simulink model "gm_fourxfour_designfxdpt_givens_vnl"  (R2018b)
settings: Solver=FixedStepDiscrete  StartTime=0.0  StopTime=0.18e-6  RelTol=1e-3
InitFcn:
  | if isempty(which('mylib'))
  |      tmp = fileparts(which(bdroot));
  |      run(fullfile(fileparts(tmp), '5-Utilities', 'addPathsPfcHw.m'));
  | end
  | 
  | data_types_givens
StopFcn:
  | GivensSim_Stop
undefined symbols (not defined in the file or in its folder): f
libraries: simulink x28, mylib x14
(part 3 of 4)

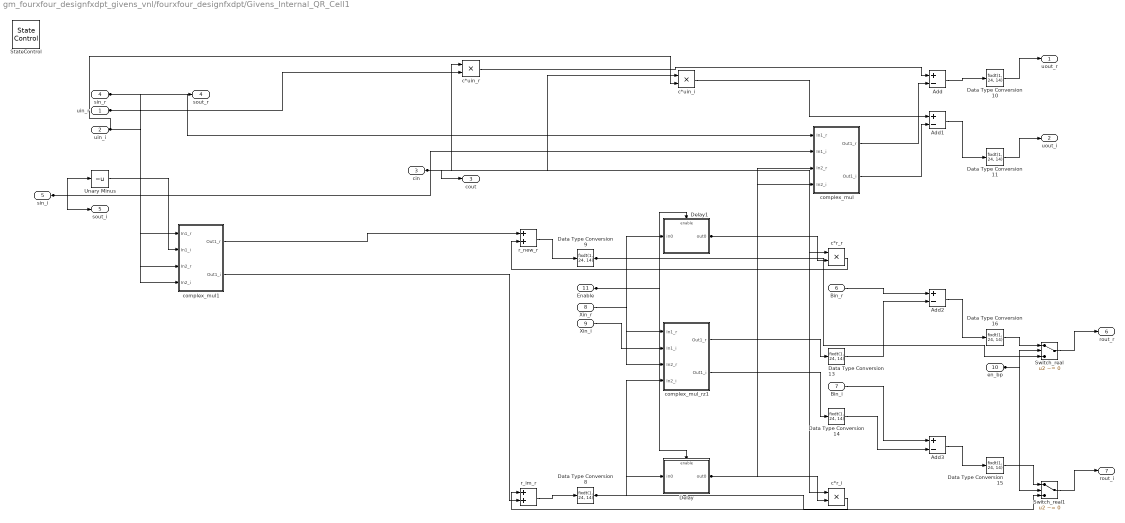
== system gm_fourxfour_designfxdpt_givens_vnl/fourxfour_designfxdpt/Givens_Internal_QR_Cell1 ==
  uin_r : Inport  OutDataTypeStr=fixdt(1, 24, 14)  SampleTime=1e-08
  uin_i : Inport  Port=2  OutDataTypeStr=fixdt(1, 24, 14)  SampleTime=1e-08
  cin : Inport  Port=3  OutDataTypeStr=fixdt(1, 24, 14)  SampleTime=1e-08
  sin_r : Inport  Port=4  OutDataTypeStr=fixdt(1, 24, 14)  SampleTime=1e-08
  sin_i : Inport  Port=5  OutDataTypeStr=fixdt(1, 24, 14)  SampleTime=1e-08
  Bin_r : Inport  Port=6  OutDataTypeStr=fixdt(1, 24, 14)  SampleTime=1e-08
  Bin_i : Inport  Port=7  OutDataTypeStr=fixdt(1, 24, 14)  SampleTime=1e-08
  Xin_r : Inport  Port=8  OutDataTypeStr=fixdt(1, 24, 14)  SampleTime=1e-08
  Xin_i : Inport  Port=9  OutDataTypeStr=fixdt(1, 24, 14)  SampleTime=1e-08
  en_bp : Inport  Port=10  OutDataTypeStr=boolean  SampleTime=1e-08
  Enable : Inport  Port=11  OutDataTypeStr=boolean  SampleTime=1e-08
  Add : Sum  Inputs=+-  AccumDataTypeStr=fixdt(1, 50, 28)  OutDataTypeStr=fixdt(1, 50, 28)  SampleTime=1e-08
  Add1 : Sum  Inputs=+-  AccumDataTypeStr=fixdt(1, 50, 28)  OutDataTypeStr=fixdt(1, 50, 28)  SampleTime=1e-08
  Add2 : Sum  Inputs=+-  AccumDataTypeStr=fixdt(1, 25, 14)  OutDataTypeStr=fixdt(1, 25, 14)  SampleTime=1e-08
  Add3 : Sum  Inputs=+-  AccumDataTypeStr=fixdt(1, 25, 14)  OutDataTypeStr=fixdt(1, 25, 14)  SampleTime=1e-08
  Data Type Conversion{8..11,13..16} (8 alike) : DataTypeConversion  OutDataTypeStr=fixdt(1, 24, 14)  SampleTime=1e-08
  Delay : Subsystem
      settings: MinAlgLoopOccurrences=on
  Delay1 : Subsystem
      settings: MinAlgLoopOccurrences=on
  StateControl : StateControl  StateControl=Synchronous
  Switch_real : Switch  Criteria=u2 ~= 0  Threshold=double(0)  OutDataTypeStr=fixdt(1, 24, 14)  SampleTime=1e-08
  Switch_real1 : Switch  Criteria=u2 ~= 0  Threshold=double(0)  OutDataTypeStr=fixdt(1, 24, 14)  SampleTime=1e-08
  Unary Minus : UnaryMinus  SampleTime=1e-08
  c*r_i : Product  Inputs=**  OutDataTypeStr=fixdt(1, 48, 28)  SampleTime=1e-08
  c*r_r : Product  Inputs=**  OutDataTypeStr=fixdt(1, 48, 28)  SampleTime=1e-08
  c*uin_i : Product  Inputs=**  OutDataTypeStr=fixdt(1, 48, 28)  SampleTime=1e-08
  c*uin_r : Product  Inputs=**  OutDataTypeStr=fixdt(1, 48, 28)  SampleTime=1e-08
  complex_mul : Subsystem
  complex_mul1 : Subsystem
  complex_mul_rz1 : Subsystem
  r_im_r : Sum  AccumDataTypeStr=fixdt(1, 50, 28)  OutDataTypeStr=fixdt(1, 50, 28)  SampleTime=1e-08
  r_new_r : Sum  AccumDataTypeStr=fixdt(1, 50, 28)  OutDataTypeStr=fixdt(1, 50, 28)  SampleTime=1e-08
  uout_r : Outport  InitialOutput=0
  uout_i : Outport  Port=2  InitialOutput=0
  cout : Outport  Port=3  InitialOutput=0
  sout_r : Outport  Port=4  InitialOutput=0
  sout_i : Outport  Port=5  InitialOutput=0
  rout_r : Outport  Port=6  InitialOutput=0
  rout_i : Outport  Port=7  InitialOutput=0
  wires:
  r_new_r/1 -> Data Type Conversion9/1
  r_im_r/1 -> Data Type Conversion8/1
  complex_mul_rz1/2(Out1_i) -> Data Type Conversion14/1
  complex_mul_rz1/1(Out1_r) -> Data Type Conversion13/1
  complex_mul1/2(Out1_i) -> r_im_r/2
  complex_mul1/1(Out1_r) -> r_new_r/1
  complex_mul/2(Out1_i) -> Add1/2
  complex_mul/1(Out1_r) -> Add/2
  c*uin_r/1 -> Add/1
  c*uin_i/1 -> Add1/1
  c*r_r/1 -> r_new_r/2
  c*r_i/1 -> r_im_r/1
  Unary Minus/1 -> complex_mul1/2(In1_i)
  Switch_real1/1 -> rout_i/1
  Switch_real/1 -> rout_r/1
  Delay1/1(out0) -> complex_mul/3(In2_r), c*r_r/2
  Delay/1(out0) -> complex_mul/4(In2_i), c*r_i/2
  Data Type Conversion9/1 -> complex_mul_rz1/3(In2_r), Delay1/1(in0), Switch_real/3
  Data Type Conversion8/1 -> complex_mul_rz1/4(In2_i), Delay/1(in0), Switch_real1/3
  Data Type Conversion16/1 -> Switch_real/1
  Data Type Conversion15/1 -> Switch_real1/1
  Data Type Conversion14/1 -> Add3/2
  Data Type Conversion13/1 -> Add2/2
  Data Type Conversion11/1 -> uout_i/1
  Data Type Conversion10/1 -> uout_r/1
  Add3/1 -> Data Type Conversion15/1
  Add2/1 -> Data Type Conversion16/1
  Add1/1 -> Data Type Conversion11/1
  Add/1 -> Data Type Conversion10/1
  en_bp/1 -> Switch_real/2, Switch_real1/2
  Xin_i/1 -> complex_mul_rz1/2(In1_i)
  Xin_r/1 -> complex_mul_rz1/1(In1_r)
  Bin_i/1 -> Add3/1
  Bin_r/1 -> Add2/1
  sin_i/1 -> sout_i/1, complex_mul/2(In1_i), Unary Minus/1
  sin_r/1 -> sout_r/1, complex_mul1/1(In1_r), complex_mul/1(In1_r)
  cin/1 -> cout/1, c*r_i/1, c*r_r/1, c*uin_i/1, c*uin_r/1
  uin_i/1 -> complex_mul1/4(In2_i), c*uin_i/2
  uin_r/1 -> complex_mul1/3(In2_r), c*uin_r/2
  Enable/1 -> Delay/Enable, Delay1/Enable

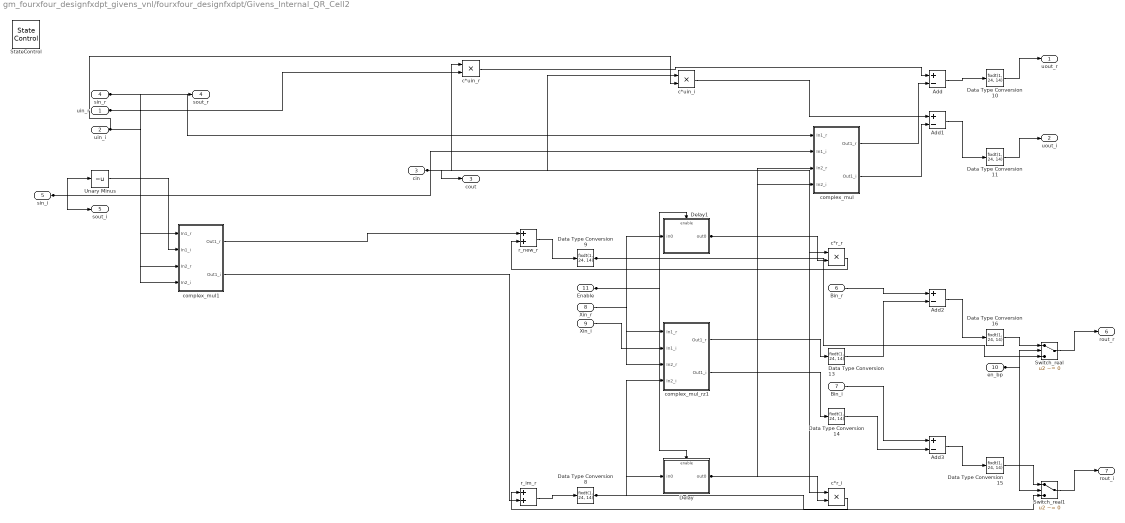
== system gm_fourxfour_designfxdpt_givens_vnl/fourxfour_designfxdpt/Givens_Internal_QR_Cell2 ==
  uin_r : Inport  OutDataTypeStr=fixdt(1, 24, 14)  SampleTime=1e-08
  uin_i : Inport  Port=2  OutDataTypeStr=fixdt(1, 24, 14)  SampleTime=1e-08
  cin : Inport  Port=3  OutDataTypeStr=fixdt(1, 24, 14)  SampleTime=1e-08
  sin_r : Inport  Port=4  OutDataTypeStr=fixdt(1, 24, 14)  SampleTime=1e-08
  sin_i : Inport  Port=5  OutDataTypeStr=fixdt(1, 24, 14)  SampleTime=1e-08
  Bin_r : Inport  Port=6  OutDataTypeStr=fixdt(1, 24, 14)  SampleTime=1e-08
  Bin_i : Inport  Port=7  OutDataTypeStr=fixdt(1, 24, 14)  SampleTime=1e-08
  Xin_r : Inport  Port=8  OutDataTypeStr=fixdt(1, 24, 14)  SampleTime=1e-08
  Xin_i : Inport  Port=9  OutDataTypeStr=fixdt(1, 24, 14)  SampleTime=1e-08
  en_bp : Inport  Port=10  OutDataTypeStr=boolean  SampleTime=1e-08
  Enable : Inport  Port=11  OutDataTypeStr=boolean  SampleTime=1e-08
  Add : Sum  Inputs=+-  AccumDataTypeStr=fixdt(1, 50, 28)  OutDataTypeStr=fixdt(1, 50, 28)  SampleTime=1e-08
  Add1 : Sum  Inputs=+-  AccumDataTypeStr=fixdt(1, 50, 28)  OutDataTypeStr=fixdt(1, 50, 28)  SampleTime=1e-08
  Add2 : Sum  Inputs=+-  AccumDataTypeStr=fixdt(1, 25, 14)  OutDataTypeStr=fixdt(1, 25, 14)  SampleTime=1e-08
  Add3 : Sum  Inputs=+-  AccumDataTypeStr=fixdt(1, 25, 14)  OutDataTypeStr=fixdt(1, 25, 14)  SampleTime=1e-08
  Data Type Conversion{8..11,13..16} (8 alike) : DataTypeConversion  OutDataTypeStr=fixdt(1, 24, 14)  SampleTime=1e-08
  Delay : Subsystem
      settings: MinAlgLoopOccurrences=on
  Delay1 : Subsystem
      settings: MinAlgLoopOccurrences=on
  StateControl : StateControl  StateControl=Synchronous
  Switch_real : Switch  Criteria=u2 ~= 0  Threshold=double(0)  OutDataTypeStr=fixdt(1, 24, 14)  SampleTime=1e-08
  Switch_real1 : Switch  Criteria=u2 ~= 0  Threshold=double(0)  OutDataTypeStr=fixdt(1, 24, 14)  SampleTime=1e-08
  Unary Minus : UnaryMinus  SampleTime=1e-08
  c*r_i : Product  Inputs=**  OutDataTypeStr=fixdt(1, 48, 28)  SampleTime=1e-08
  c*r_r : Product  Inputs=**  OutDataTypeStr=fixdt(1, 48, 28)  SampleTime=1e-08
  c*uin_i : Product  Inputs=**  OutDataTypeStr=fixdt(1, 48, 28)  SampleTime=1e-08
  c*uin_r : Product  Inputs=**  OutDataTypeStr=fixdt(1, 48, 28)  SampleTime=1e-08
  complex_mul : Subsystem
  complex_mul1 : Subsystem
  complex_mul_rz1 : Subsystem
  r_im_r : Sum  AccumDataTypeStr=fixdt(1, 50, 28)  OutDataTypeStr=fixdt(1, 50, 28)  SampleTime=1e-08
  r_new_r : Sum  AccumDataTypeStr=fixdt(1, 50, 28)  OutDataTypeStr=fixdt(1, 50, 28)  SampleTime=1e-08
  uout_r : Outport  InitialOutput=0
  uout_i : Outport  Port=2  InitialOutput=0
  cout : Outport  Port=3  InitialOutput=0
  sout_r : Outport  Port=4  InitialOutput=0
  sout_i : Outport  Port=5  InitialOutput=0
  rout_r : Outport  Port=6  InitialOutput=0
  rout_i : Outport  Port=7  InitialOutput=0
  wires:
  r_new_r/1 -> Data Type Conversion9/1
  r_im_r/1 -> Data Type Conversion8/1
  complex_mul_rz1/2(Out1_i) -> Data Type Conversion14/1
  complex_mul_rz1/1(Out1_r) -> Data Type Conversion13/1
  complex_mul1/2(Out1_i) -> r_im_r/2
  complex_mul1/1(Out1_r) -> r_new_r/1
  complex_mul/2(Out1_i) -> Add1/2
  complex_mul/1(Out1_r) -> Add/2
  c*uin_r/1 -> Add/1
  c*uin_i/1 -> Add1/1
  c*r_r/1 -> r_new_r/2
  c*r_i/1 -> r_im_r/1
  Unary Minus/1 -> complex_mul1/2(In1_i)
  Switch_real1/1 -> rout_i/1
  Switch_real/1 -> rout_r/1
  Delay1/1(out0) -> complex_mul/3(In2_r), c*r_r/2
  Delay/1(out0) -> complex_mul/4(In2_i), c*r_i/2
  Data Type Conversion9/1 -> complex_mul_rz1/3(In2_r), Delay1/1(in0), Switch_real/3
  Data Type Conversion8/1 -> complex_mul_rz1/4(In2_i), Delay/1(in0), Switch_real1/3
  Data Type Conversion16/1 -> Switch_real/1
  Data Type Conversion15/1 -> Switch_real1/1
  Data Type Conversion14/1 -> Add3/2
  Data Type Conversion13/1 -> Add2/2
  Data Type Conversion11/1 -> uout_i/1
  Data Type Conversion10/1 -> uout_r/1
  Add3/1 -> Data Type Conversion15/1
  Add2/1 -> Data Type Conversion16/1
  Add1/1 -> Data Type Conversion11/1
  Add/1 -> Data Type Conversion10/1
  en_bp/1 -> Switch_real/2, Switch_real1/2
  Xin_i/1 -> complex_mul_rz1/2(In1_i)
  Xin_r/1 -> complex_mul_rz1/1(In1_r)
  Bin_i/1 -> Add3/1
  Bin_r/1 -> Add2/1
  sin_i/1 -> sout_i/1, complex_mul/2(In1_i), Unary Minus/1
  sin_r/1 -> sout_r/1, complex_mul1/1(In1_r), complex_mul/1(In1_r)
  cin/1 -> cout/1, c*r_i/1, c*r_r/1, c*uin_i/1, c*uin_r/1
  uin_i/1 -> complex_mul1/4(In2_i), c*uin_i/2
  uin_r/1 -> complex_mul1/3(In2_r), c*uin_r/2
  Enable/1 -> Delay/Enable, Delay1/Enable

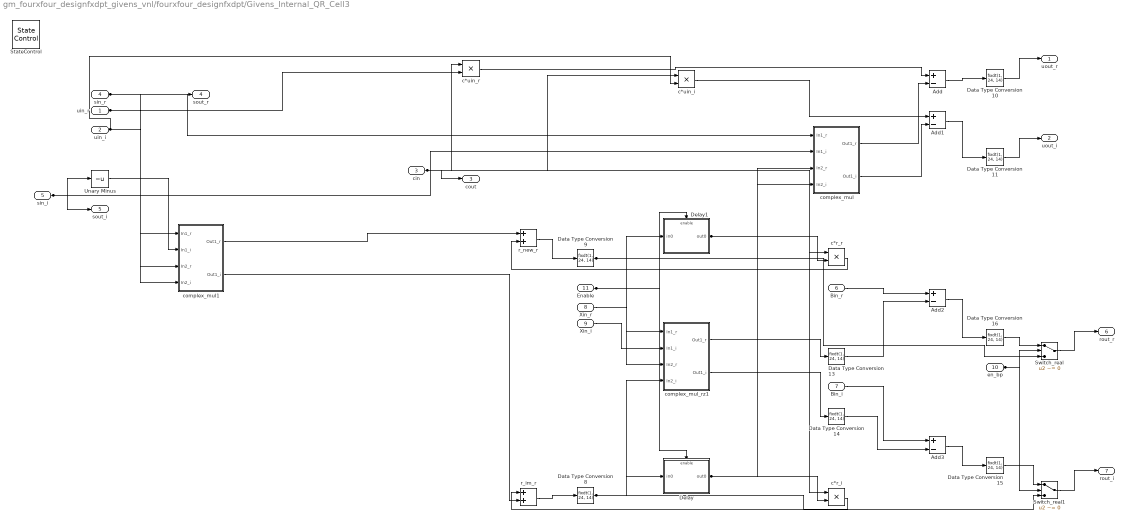
== system gm_fourxfour_designfxdpt_givens_vnl/fourxfour_designfxdpt/Givens_Internal_QR_Cell3 ==
  uin_r : Inport  OutDataTypeStr=fixdt(1, 24, 14)  SampleTime=1e-08
  uin_i : Inport  Port=2  OutDataTypeStr=fixdt(1, 24, 14)  SampleTime=1e-08
  cin : Inport  Port=3  OutDataTypeStr=fixdt(1, 24, 14)  SampleTime=1e-08
  sin_r : Inport  Port=4  OutDataTypeStr=fixdt(1, 24, 14)  SampleTime=1e-08
  sin_i : Inport  Port=5  OutDataTypeStr=fixdt(1, 24, 14)  SampleTime=1e-08
  Bin_r : Inport  Port=6  OutDataTypeStr=fixdt(1, 24, 14)  SampleTime=1e-08
  Bin_i : Inport  Port=7  OutDataTypeStr=fixdt(1, 24, 14)  SampleTime=1e-08
  Xin_r : Inport  Port=8  OutDataTypeStr=fixdt(1, 24, 14)  SampleTime=1e-08
  Xin_i : Inport  Port=9  OutDataTypeStr=fixdt(1, 24, 14)  SampleTime=1e-08
  en_bp : Inport  Port=10  OutDataTypeStr=boolean  SampleTime=1e-08
  Enable : Inport  Port=11  OutDataTypeStr=boolean  SampleTime=1e-08
  Add : Sum  Inputs=+-  AccumDataTypeStr=fixdt(1, 50, 28)  OutDataTypeStr=fixdt(1, 50, 28)  SampleTime=1e-08
  Add1 : Sum  Inputs=+-  AccumDataTypeStr=fixdt(1, 50, 28)  OutDataTypeStr=fixdt(1, 50, 28)  SampleTime=1e-08
  Add2 : Sum  Inputs=+-  AccumDataTypeStr=fixdt(1, 25, 14)  OutDataTypeStr=fixdt(1, 25, 14)  SampleTime=1e-08
  Add3 : Sum  Inputs=+-  AccumDataTypeStr=fixdt(1, 25, 14)  OutDataTypeStr=fixdt(1, 25, 14)  SampleTime=1e-08
  Data Type Conversion{8..11,13..16} (8 alike) : DataTypeConversion  OutDataTypeStr=fixdt(1, 24, 14)  SampleTime=1e-08
  Delay : Subsystem
      settings: MinAlgLoopOccurrences=on
  Delay1 : Subsystem
      settings: MinAlgLoopOccurrences=on
  StateControl : StateControl  StateControl=Synchronous
  Switch_real : Switch  Criteria=u2 ~= 0  Threshold=double(0)  OutDataTypeStr=fixdt(1, 24, 14)  SampleTime=1e-08
  Switch_real1 : Switch  Criteria=u2 ~= 0  Threshold=double(0)  OutDataTypeStr=fixdt(1, 24, 14)  SampleTime=1e-08
  Unary Minus : UnaryMinus  SampleTime=1e-08
  c*r_i : Product  Inputs=**  OutDataTypeStr=fixdt(1, 48, 28)  SampleTime=1e-08
  c*r_r : Product  Inputs=**  OutDataTypeStr=fixdt(1, 48, 28)  SampleTime=1e-08
  c*uin_i : Product  Inputs=**  OutDataTypeStr=fixdt(1, 48, 28)  SampleTime=1e-08
  c*uin_r : Product  Inputs=**  OutDataTypeStr=fixdt(1, 48, 28)  SampleTime=1e-08
  complex_mul : Subsystem
  complex_mul1 : Subsystem
  complex_mul_rz1 : Subsystem
  r_im_r : Sum  AccumDataTypeStr=fixdt(1, 50, 28)  OutDataTypeStr=fixdt(1, 50, 28)  SampleTime=1e-08
  r_new_r : Sum  AccumDataTypeStr=fixdt(1, 50, 28)  OutDataTypeStr=fixdt(1, 50, 28)  SampleTime=1e-08
  uout_r : Outport  InitialOutput=0
  uout_i : Outport  Port=2  InitialOutput=0
  cout : Outport  Port=3  InitialOutput=0
  sout_r : Outport  Port=4  InitialOutput=0
  sout_i : Outport  Port=5  InitialOutput=0
  rout_r : Outport  Port=6  InitialOutput=0
  rout_i : Outport  Port=7  InitialOutput=0
  wires:
  r_new_r/1 -> Data Type Conversion9/1
  r_im_r/1 -> Data Type Conversion8/1
  complex_mul_rz1/2(Out1_i) -> Data Type Conversion14/1
  complex_mul_rz1/1(Out1_r) -> Data Type Conversion13/1
  complex_mul1/2(Out1_i) -> r_im_r/2
  complex_mul1/1(Out1_r) -> r_new_r/1
  complex_mul/2(Out1_i) -> Add1/2
  complex_mul/1(Out1_r) -> Add/2
  c*uin_r/1 -> Add/1
  c*uin_i/1 -> Add1/1
  c*r_r/1 -> r_new_r/2
  c*r_i/1 -> r_im_r/1
  Unary Minus/1 -> complex_mul1/2(In1_i)
  Switch_real1/1 -> rout_i/1
  Switch_real/1 -> rout_r/1
  Delay1/1(out0) -> complex_mul/3(In2_r), c*r_r/2
  Delay/1(out0) -> complex_mul/4(In2_i), c*r_i/2
  Data Type Conversion9/1 -> complex_mul_rz1/3(In2_r), Delay1/1(in0), Switch_real/3
  Data Type Conversion8/1 -> complex_mul_rz1/4(In2_i), Delay/1(in0), Switch_real1/3
  Data Type Conversion16/1 -> Switch_real/1
  Data Type Conversion15/1 -> Switch_real1/1
  Data Type Conversion14/1 -> Add3/2
  Data Type Conversion13/1 -> Add2/2
  Data Type Conversion11/1 -> uout_i/1
  Data Type Conversion10/1 -> uout_r/1
  Add3/1 -> Data Type Conversion15/1
  Add2/1 -> Data Type Conversion16/1
  Add1/1 -> Data Type Conversion11/1
  Add/1 -> Data Type Conversion10/1
  en_bp/1 -> Switch_real/2, Switch_real1/2
  Xin_i/1 -> complex_mul_rz1/2(In1_i)
  Xin_r/1 -> complex_mul_rz1/1(In1_r)
  Bin_i/1 -> Add3/1
  Bin_r/1 -> Add2/1
  sin_i/1 -> sout_i/1, complex_mul/2(In1_i), Unary Minus/1
  sin_r/1 -> sout_r/1, complex_mul1/1(In1_r), complex_mul/1(In1_r)
  cin/1 -> cout/1, c*r_i/1, c*r_r/1, c*uin_i/1, c*uin_r/1
  uin_i/1 -> complex_mul1/4(In2_i), c*uin_i/2
  uin_r/1 -> complex_mul1/3(In2_r), c*uin_r/2
  Enable/1 -> Delay/Enable, Delay1/Enable

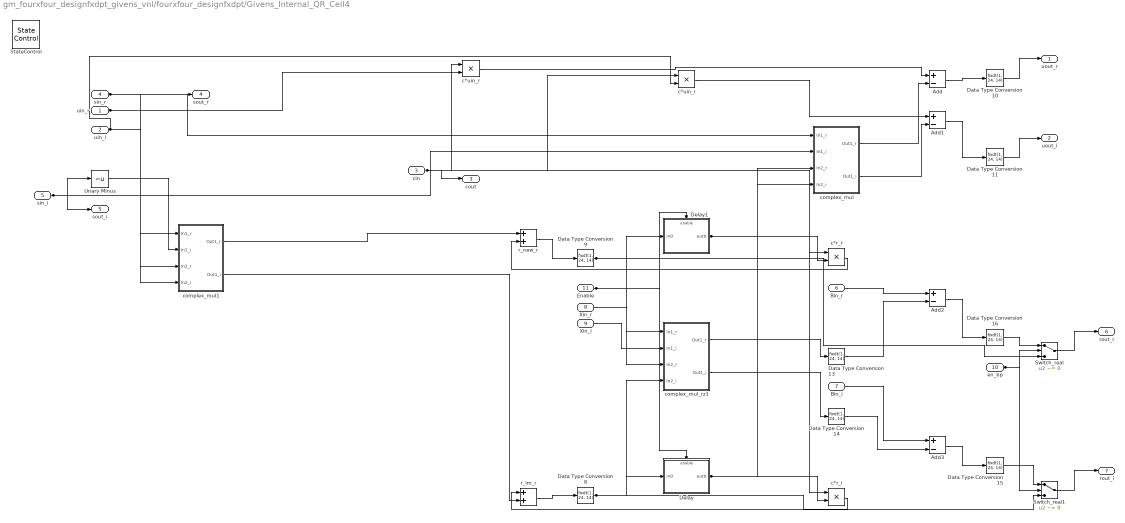
== system gm_fourxfour_designfxdpt_givens_vnl/fourxfour_designfxdpt/Givens_Internal_QR_Cell4 ==
  uin_r : Inport  OutDataTypeStr=fixdt(1, 24, 14)  SampleTime=1e-08
  uin_i : Inport  Port=2  OutDataTypeStr=fixdt(1, 24, 14)  SampleTime=1e-08
  cin : Inport  Port=3  OutDataTypeStr=fixdt(1, 24, 14)  SampleTime=1e-08
  sin_r : Inport  Port=4  OutDataTypeStr=fixdt(1, 24, 14)  SampleTime=1e-08
  sin_i : Inport  Port=5  OutDataTypeStr=fixdt(1, 24, 14)  SampleTime=1e-08
  Bin_r : Inport  Port=6  OutDataTypeStr=fixdt(1, 24, 14)  SampleTime=1e-08
  Bin_i : Inport  Port=7  OutDataTypeStr=fixdt(1, 24, 14)  SampleTime=1e-08
  Xin_r : Inport  Port=8  OutDataTypeStr=fixdt(1, 24, 14)  SampleTime=1e-08
  Xin_i : Inport  Port=9  OutDataTypeStr=fixdt(1, 24, 14)  SampleTime=1e-08
  en_bp : Inport  Port=10  OutDataTypeStr=boolean  SampleTime=1e-08
  Enable : Inport  Port=11  OutDataTypeStr=boolean  SampleTime=1e-08
  Add : Sum  Inputs=+-  AccumDataTypeStr=fixdt(1, 50, 28)  OutDataTypeStr=fixdt(1, 50, 28)  SampleTime=1e-08
  Add1 : Sum  Inputs=+-  AccumDataTypeStr=fixdt(1, 50, 28)  OutDataTypeStr=fixdt(1, 50, 28)  SampleTime=1e-08
  Add2 : Sum  Inputs=+-  AccumDataTypeStr=fixdt(1, 25, 14)  OutDataTypeStr=fixdt(1, 25, 14)  SampleTime=1e-08
  Add3 : Sum  Inputs=+-  AccumDataTypeStr=fixdt(1, 25, 14)  OutDataTypeStr=fixdt(1, 25, 14)  SampleTime=1e-08
  Data Type Conversion{8..11,13..16} (8 alike) : DataTypeConversion  OutDataTypeStr=fixdt(1, 24, 14)  SampleTime=1e-08
  Delay : Subsystem
      settings: MinAlgLoopOccurrences=on
  Delay1 : Subsystem
      settings: MinAlgLoopOccurrences=on
  StateControl : StateControl  StateControl=Synchronous
  Switch_real : Switch  Criteria=u2 ~= 0  Threshold=double(0)  OutDataTypeStr=fixdt(1, 24, 14)  SampleTime=1e-08
  Switch_real1 : Switch  Criteria=u2 ~= 0  Threshold=double(0)  OutDataTypeStr=fixdt(1, 24, 14)  SampleTime=1e-08
  Unary Minus : UnaryMinus  SampleTime=1e-08
  c*r_i : Product  Inputs=**  OutDataTypeStr=fixdt(1, 48, 28)  SampleTime=1e-08
  c*r_r : Product  Inputs=**  OutDataTypeStr=fixdt(1, 48, 28)  SampleTime=1e-08
  c*uin_i : Product  Inputs=**  OutDataTypeStr=fixdt(1, 48, 28)  SampleTime=1e-08
  c*uin_r : Product  Inputs=**  OutDataTypeStr=fixdt(1, 48, 28)  SampleTime=1e-08
  complex_mul : Subsystem
  complex_mul1 : Subsystem
  complex_mul_rz1 : Subsystem
  r_im_r : Sum  AccumDataTypeStr=fixdt(1, 50, 28)  OutDataTypeStr=fixdt(1, 50, 28)  SampleTime=1e-08
  r_new_r : Sum  AccumDataTypeStr=fixdt(1, 50, 28)  OutDataTypeStr=fixdt(1, 50, 28)  SampleTime=1e-08
  uout_r : Outport  InitialOutput=0
  uout_i : Outport  Port=2  InitialOutput=0
  cout : Outport  Port=3  InitialOutput=0
  sout_r : Outport  Port=4  InitialOutput=0
  sout_i : Outport  Port=5  InitialOutput=0
  rout_r : Outport  Port=6  InitialOutput=0
  rout_i : Outport  Port=7  InitialOutput=0
  wires:
  r_new_r/1 -> Data Type Conversion9/1
  r_im_r/1 -> Data Type Conversion8/1
  complex_mul_rz1/2(Out1_i) -> Data Type Conversion14/1
  complex_mul_rz1/1(Out1_r) -> Data Type Conversion13/1
  complex_mul1/2(Out1_i) -> r_im_r/2
  complex_mul1/1(Out1_r) -> r_new_r/1
  complex_mul/2(Out1_i) -> Add1/2
  complex_mul/1(Out1_r) -> Add/2
  c*uin_r/1 -> Add/1
  c*uin_i/1 -> Add1/1
  c*r_r/1 -> r_new_r/2
  c*r_i/1 -> r_im_r/1
  Unary Minus/1 -> complex_mul1/2(In1_i)
  Switch_real1/1 -> rout_i/1
  Switch_real/1 -> rout_r/1
  Delay1/1(out0) -> complex_mul/3(In2_r), c*r_r/2
  Delay/1(out0) -> complex_mul/4(In2_i), c*r_i/2
  Data Type Conversion9/1 -> complex_mul_rz1/3(In2_r), Delay1/1(in0), Switch_real/3
  Data Type Conversion8/1 -> complex_mul_rz1/4(In2_i), Delay/1(in0), Switch_real1/3
  Data Type Conversion16/1 -> Switch_real/1
  Data Type Conversion15/1 -> Switch_real1/1
  Data Type Conversion14/1 -> Add3/2
  Data Type Conversion13/1 -> Add2/2
  Data Type Conversion11/1 -> uout_i/1
  Data Type Conversion10/1 -> uout_r/1
  Add3/1 -> Data Type Conversion15/1
  Add2/1 -> Data Type Conversion16/1
  Add1/1 -> Data Type Conversion11/1
  Add/1 -> Data Type Conversion10/1
  en_bp/1 -> Switch_real/2, Switch_real1/2
  Xin_i/1 -> complex_mul_rz1/2(In1_i)
  Xin_r/1 -> complex_mul_rz1/1(In1_r)
  Bin_i/1 -> Add3/1
  Bin_r/1 -> Add2/1
  sin_i/1 -> sout_i/1, complex_mul/2(In1_i), Unary Minus/1
  sin_r/1 -> sout_r/1, complex_mul1/1(In1_r), complex_mul/1(In1_r)
  cin/1 -> cout/1, c*r_i/1, c*r_r/1, c*uin_i/1, c*uin_r/1
  uin_i/1 -> complex_mul1/4(In2_i), c*uin_i/2
  uin_r/1 -> complex_mul1/3(In2_r), c*uin_r/2
  Enable/1 -> Delay/Enable, Delay1/Enable

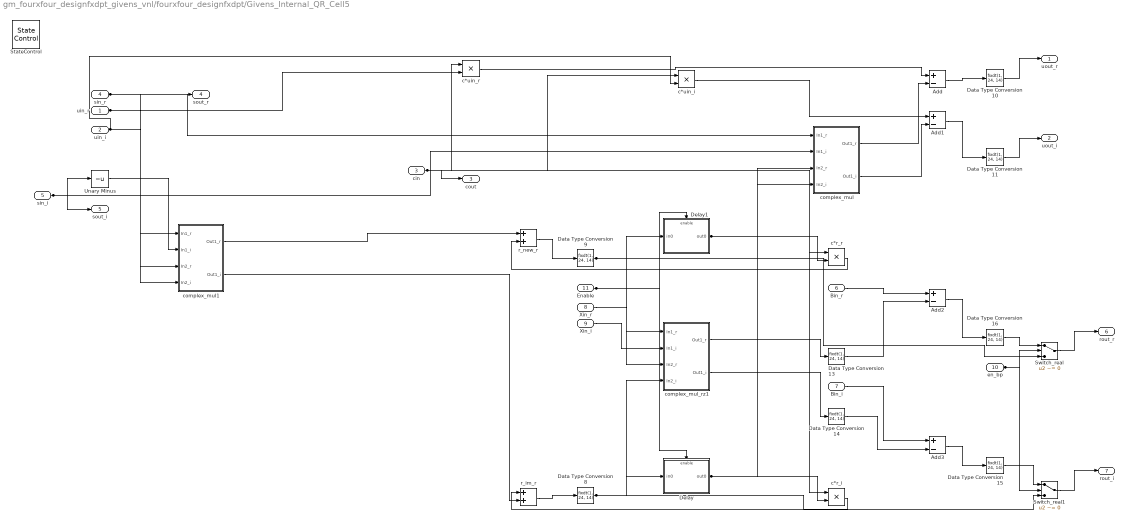
== system gm_fourxfour_designfxdpt_givens_vnl/fourxfour_designfxdpt/Givens_Internal_QR_Cell5 ==
  uin_r : Inport  OutDataTypeStr=fixdt(1, 24, 14)  SampleTime=1e-08
  uin_i : Inport  Port=2  OutDataTypeStr=fixdt(1, 24, 14)  SampleTime=1e-08
  cin : Inport  Port=3  OutDataTypeStr=fixdt(1, 24, 14)  SampleTime=1e-08
  sin_r : Inport  Port=4  OutDataTypeStr=fixdt(1, 24, 14)  SampleTime=1e-08
  sin_i : Inport  Port=5  OutDataTypeStr=fixdt(1, 24, 14)  SampleTime=1e-08
  Bin_r : Inport  Port=6  OutDataTypeStr=fixdt(1, 24, 14)  SampleTime=1e-08
  Bin_i : Inport  Port=7  OutDataTypeStr=fixdt(1, 24, 14)  SampleTime=1e-08
  Xin_r : Inport  Port=8  OutDataTypeStr=fixdt(1, 24, 14)  SampleTime=1e-08
  Xin_i : Inport  Port=9  OutDataTypeStr=fixdt(1, 24, 14)  SampleTime=1e-08
  en_bp : Inport  Port=10  OutDataTypeStr=boolean  SampleTime=1e-08
  Enable : Inport  Port=11  OutDataTypeStr=boolean  SampleTime=1e-08
  Add : Sum  Inputs=+-  AccumDataTypeStr=fixdt(1, 50, 28)  OutDataTypeStr=fixdt(1, 50, 28)  SampleTime=1e-08
  Add1 : Sum  Inputs=+-  AccumDataTypeStr=fixdt(1, 50, 28)  OutDataTypeStr=fixdt(1, 50, 28)  SampleTime=1e-08
  Add2 : Sum  Inputs=+-  AccumDataTypeStr=fixdt(1, 25, 14)  OutDataTypeStr=fixdt(1, 25, 14)  SampleTime=1e-08
  Add3 : Sum  Inputs=+-  AccumDataTypeStr=fixdt(1, 25, 14)  OutDataTypeStr=fixdt(1, 25, 14)  SampleTime=1e-08
  Data Type Conversion{8..11,13..16} (8 alike) : DataTypeConversion  OutDataTypeStr=fixdt(1, 24, 14)  SampleTime=1e-08
  Delay : Subsystem
      settings: MinAlgLoopOccurrences=on
  Delay1 : Subsystem
      settings: MinAlgLoopOccurrences=on
  StateControl : StateControl  StateControl=Synchronous
  Switch_real : Switch  Criteria=u2 ~= 0  Threshold=double(0)  OutDataTypeStr=fixdt(1, 24, 14)  SampleTime=1e-08
  Switch_real1 : Switch  Criteria=u2 ~= 0  Threshold=double(0)  OutDataTypeStr=fixdt(1, 24, 14)  SampleTime=1e-08
  Unary Minus : UnaryMinus  SampleTime=1e-08
  c*r_i : Product  Inputs=**  OutDataTypeStr=fixdt(1, 48, 28)  SampleTime=1e-08
  c*r_r : Product  Inputs=**  OutDataTypeStr=fixdt(1, 48, 28)  SampleTime=1e-08
  c*uin_i : Product  Inputs=**  OutDataTypeStr=fixdt(1, 48, 28)  SampleTime=1e-08
  c*uin_r : Product  Inputs=**  OutDataTypeStr=fixdt(1, 48, 28)  SampleTime=1e-08
  complex_mul : Subsystem
  complex_mul1 : Subsystem
  complex_mul_rz1 : Subsystem
  r_im_r : Sum  AccumDataTypeStr=fixdt(1, 50, 28)  OutDataTypeStr=fixdt(1, 50, 28)  SampleTime=1e-08
  r_new_r : Sum  AccumDataTypeStr=fixdt(1, 50, 28)  OutDataTypeStr=fixdt(1, 50, 28)  SampleTime=1e-08
  uout_r : Outport  InitialOutput=0
  uout_i : Outport  Port=2  InitialOutput=0
  cout : Outport  Port=3  InitialOutput=0
  sout_r : Outport  Port=4  InitialOutput=0
  sout_i : Outport  Port=5  InitialOutput=0
  rout_r : Outport  Port=6  InitialOutput=0
  rout_i : Outport  Port=7  InitialOutput=0
  wires:
  r_new_r/1 -> Data Type Conversion9/1
  r_im_r/1 -> Data Type Conversion8/1
  complex_mul_rz1/2(Out1_i) -> Data Type Conversion14/1
  complex_mul_rz1/1(Out1_r) -> Data Type Conversion13/1
  complex_mul1/2(Out1_i) -> r_im_r/2
  complex_mul1/1(Out1_r) -> r_new_r/1
  complex_mul/2(Out1_i) -> Add1/2
  complex_mul/1(Out1_r) -> Add/2
  c*uin_r/1 -> Add/1
  c*uin_i/1 -> Add1/1
  c*r_r/1 -> r_new_r/2
  c*r_i/1 -> r_im_r/1
  Unary Minus/1 -> complex_mul1/2(In1_i)
  Switch_real1/1 -> rout_i/1
  Switch_real/1 -> rout_r/1
  Delay1/1(out0) -> complex_mul/3(In2_r), c*r_r/2
  Delay/1(out0) -> complex_mul/4(In2_i), c*r_i/2
  Data Type Conversion9/1 -> complex_mul_rz1/3(In2_r), Delay1/1(in0), Switch_real/3
  Data Type Conversion8/1 -> complex_mul_rz1/4(In2_i), Delay/1(in0), Switch_real1/3
  Data Type Conversion16/1 -> Switch_real/1
  Data Type Conversion15/1 -> Switch_real1/1
  Data Type Conversion14/1 -> Add3/2
  Data Type Conversion13/1 -> Add2/2
  Data Type Conversion11/1 -> uout_i/1
  Data Type Conversion10/1 -> uout_r/1
  Add3/1 -> Data Type Conversion15/1
  Add2/1 -> Data Type Conversion16/1
  Add1/1 -> Data Type Conversion11/1
  Add/1 -> Data Type Conversion10/1
  en_bp/1 -> Switch_real/2, Switch_real1/2
  Xin_i/1 -> complex_mul_rz1/2(In1_i)
  Xin_r/1 -> complex_mul_rz1/1(In1_r)
  Bin_i/1 -> Add3/1
  Bin_r/1 -> Add2/1
  sin_i/1 -> sout_i/1, complex_mul/2(In1_i), Unary Minus/1
  sin_r/1 -> sout_r/1, complex_mul1/1(In1_r), complex_mul/1(In1_r)
  cin/1 -> cout/1, c*r_i/1, c*r_r/1, c*uin_i/1, c*uin_r/1
  uin_i/1 -> complex_mul1/4(In2_i), c*uin_i/2
  uin_r/1 -> complex_mul1/3(In2_r), c*uin_r/2
  Enable/1 -> Delay/Enable, Delay1/Enable

== system gm_fourxfour_designfxdpt_givens_vnl/fourxfour_designfxdpt/Givens_Boundary_Cell/Delay1 ==
  in0 : Inport  OutDataTypeStr=fixdt(1, 48, 28)  SampleTime=1e-08
  Enable_out6 : EnablePort  OutDataTypeStr=boolean
  Delay1 : Delay  DelayLength=double(1)  InitialCondition=0  InputProcessing=Inherited
  out0 : Outport  OutDataTypeStr=fixdt(1, 48, 28)  InitialOutput=0
  wires:
  in0/1 -> Delay1/1
  Delay1/1 -> out0/1

== system gm_fourxfour_designfxdpt_givens_vnl/fourxfour_designfxdpt/Givens_Boundary_Cell/Delay2 ==
  in0 : Inport  OutDataTypeStr=fixdt(1, 24, 14)  SampleTime=1e-08
  Enable_out6 : EnablePort  OutDataTypeStr=boolean
  Delay2 : Delay  DelayLength=double(4)  InitialCondition=0  InputProcessing=Inherited
  out0 : Outport  OutDataTypeStr=fixdt(1, 24, 14)  InitialOutput=0
  wires:
  in0/1 -> Delay2/1
  Delay2/1 -> out0/1

== system gm_fourxfour_designfxdpt_givens_vnl/fourxfour_designfxdpt/Givens_Boundary_Cell/Delay3 ==
  in0 : Inport  OutDataTypeStr=fixdt(1, 24, 14)  SampleTime=1e-08
  Enable_out6 : EnablePort  OutDataTypeStr=boolean
  Delay3 : Delay  DelayLength=double(4)  InitialCondition=0  InputProcessing=Inherited
  out0 : Outport  OutDataTypeStr=fixdt(1, 24, 14)  InitialOutput=0
  wires:
  in0/1 -> Delay3/1
  Delay3/1 -> out0/1

== system gm_fourxfour_designfxdpt_givens_vnl/fourxfour_designfxdpt/Givens_Boundary_Cell/Delay4 ==
  in0 : Inport  OutDataTypeStr=fixdt(0, 49, 28)  SampleTime=1e-08
  Enable_out6 : EnablePort  OutDataTypeStr=boolean
  Delay4 : Delay  DelayLength=double(5)  InitialCondition=0  InputProcessing=Inherited
  out0 : Outport  OutDataTypeStr=fixdt(0, 49, 28)  InitialOutput=0
  wires:
  in0/1 -> Delay4/1
  Delay4/1 -> out0/1

== system gm_fourxfour_designfxdpt_givens_vnl/fourxfour_designfxdpt/Givens_Boundary_Cell/Delay5 ==
  in0 : Inport  OutDataTypeStr=fixdt(1, 73, 34)  SampleTime=1e-08
  Enable_out6 : EnablePort  OutDataTypeStr=boolean
  Delay5 : Delay  DelayLength=double(4)  InitialCondition=0  InputProcessing=Inherited
  out0 : Outport  OutDataTypeStr=fixdt(1, 73, 34)  InitialOutput=0
  wires:
  in0/1 -> Delay5/1
  Delay5/1 -> out0/1

== system gm_fourxfour_designfxdpt_givens_vnl/fourxfour_designfxdpt/Givens_Boundary_Cell/Delay6 ==
  in0 : Inport  OutDataTypeStr=fixdt(1, 73, 34)  SampleTime=1e-08
  Enable_out6 : EnablePort  OutDataTypeStr=boolean
  Delay6 : Delay  DelayLength=double(4)  InitialCondition=0  InputProcessing=Inherited
  out0 : Outport  OutDataTypeStr=fixdt(1, 73, 34)  InitialOutput=0
  wires:
  in0/1 -> Delay6/1
  Delay6/1 -> out0/1

== system gm_fourxfour_designfxdpt_givens_vnl/fourxfour_designfxdpt/Givens_Boundary_Cell/HDL Reciprocal ==
  In1 : Inport
  Delay1 : Delay  DelayLength=1  InputProcessing=Inherited
  Delay2 : Delay  DelayLength=3  InputProcessing=Inherited
  HDL Reciprocal : Reciprocal  SampleTime=1e-08
  Out1 : Outport
  wires:
  Delay2/1 -> Out1/1
  HDL Reciprocal/1 -> Delay2/1
  Delay1/1 -> HDL Reciprocal/1
  In1/1 -> Delay1/1

== system gm_fourxfour_designfxdpt_givens_vnl/fourxfour_designfxdpt/Givens_Boundary_Cell1/Delay1 ==
  in0 : Inport  OutDataTypeStr=fixdt(1, 48, 28)  SampleTime=1e-08
  Enable_out6 : EnablePort  OutDataTypeStr=boolean
  Delay1 : Delay  DelayLength=double(1)  InitialCondition=0  InputProcessing=Inherited
  out0 : Outport  OutDataTypeStr=fixdt(1, 48, 28)  InitialOutput=0
  wires:
  in0/1 -> Delay1/1
  Delay1/1 -> out0/1

== system gm_fourxfour_designfxdpt_givens_vnl/fourxfour_designfxdpt/Givens_Boundary_Cell1/Delay2 ==
  in0 : Inport  OutDataTypeStr=fixdt(1, 24, 14)  SampleTime=1e-08
  Enable_out6 : EnablePort  OutDataTypeStr=boolean
  Delay2 : Delay  DelayLength=double(4)  InitialCondition=0  InputProcessing=Inherited
  out0 : Outport  OutDataTypeStr=fixdt(1, 24, 14)  InitialOutput=0
  wires:
  in0/1 -> Delay2/1
  Delay2/1 -> out0/1

== system gm_fourxfour_designfxdpt_givens_vnl/fourxfour_designfxdpt/Givens_Boundary_Cell1/Delay3 ==
  in0 : Inport  OutDataTypeStr=fixdt(1, 24, 14)  SampleTime=1e-08
  Enable_out6 : EnablePort  OutDataTypeStr=boolean
  Delay3 : Delay  DelayLength=double(4)  InitialCondition=0  InputProcessing=Inherited
  out0 : Outport  OutDataTypeStr=fixdt(1, 24, 14)  InitialOutput=0
  wires:
  in0/1 -> Delay3/1
  Delay3/1 -> out0/1

== system gm_fourxfour_designfxdpt_givens_vnl/fourxfour_designfxdpt/Givens_Boundary_Cell1/Delay4 ==
  in0 : Inport  OutDataTypeStr=fixdt(0, 49, 28)  SampleTime=1e-08
  Enable_out6 : EnablePort  OutDataTypeStr=boolean
  Delay4 : Delay  DelayLength=double(5)  InitialCondition=0  InputProcessing=Inherited
  out0 : Outport  OutDataTypeStr=fixdt(0, 49, 28)  InitialOutput=0
  wires:
  in0/1 -> Delay4/1
  Delay4/1 -> out0/1

== system gm_fourxfour_designfxdpt_givens_vnl/fourxfour_designfxdpt/Givens_Boundary_Cell1/Delay5 ==
  in0 : Inport  OutDataTypeStr=fixdt(1, 73, 34)  SampleTime=1e-08
  Enable_out6 : EnablePort  OutDataTypeStr=boolean
  Delay5 : Delay  DelayLength=double(4)  InitialCondition=0  InputProcessing=Inherited
  out0 : Outport  OutDataTypeStr=fixdt(1, 73, 34)  InitialOutput=0
  wires:
  in0/1 -> Delay5/1
  Delay5/1 -> out0/1

== system gm_fourxfour_designfxdpt_givens_vnl/fourxfour_designfxdpt/Givens_Boundary_Cell1/Delay6 ==
  in0 : Inport  OutDataTypeStr=fixdt(1, 73, 34)  SampleTime=1e-08
  Enable_out6 : EnablePort  OutDataTypeStr=boolean
  Delay6 : Delay  DelayLength=double(4)  InitialCondition=0  InputProcessing=Inherited
  out0 : Outport  OutDataTypeStr=fixdt(1, 73, 34)  InitialOutput=0
  wires:
  in0/1 -> Delay6/1
  Delay6/1 -> out0/1

== system gm_fourxfour_designfxdpt_givens_vnl/fourxfour_designfxdpt/Givens_Boundary_Cell1/HDL Reciprocal ==
  In1 : Inport
  Delay1 : Delay  DelayLength=1  InputProcessing=Inherited
  Delay2 : Delay  DelayLength=3  InputProcessing=Inherited
  HDL Reciprocal : Reciprocal  SampleTime=1e-08
  Out1 : Outport
  wires:
  Delay2/1 -> Out1/1
  HDL Reciprocal/1 -> Delay2/1
  Delay1/1 -> HDL Reciprocal/1
  In1/1 -> Delay1/1

== system gm_fourxfour_designfxdpt_givens_vnl/fourxfour_designfxdpt/Givens_Boundary_Cell2/Delay1 ==
  in0 : Inport  OutDataTypeStr=fixdt(1, 48, 28)  SampleTime=1e-08
  Enable_out6 : EnablePort  OutDataTypeStr=boolean
  Delay1 : Delay  DelayLength=double(1)  InitialCondition=0  InputProcessing=Inherited
  out0 : Outport  OutDataTypeStr=fixdt(1, 48, 28)  InitialOutput=0
  wires:
  in0/1 -> Delay1/1
  Delay1/1 -> out0/1

== system gm_fourxfour_designfxdpt_givens_vnl/fourxfour_designfxdpt/Givens_Boundary_Cell2/Delay2 ==
  in0 : Inport  OutDataTypeStr=fixdt(1, 24, 14)  SampleTime=1e-08
  Enable_out6 : EnablePort  OutDataTypeStr=boolean
  Delay2 : Delay  DelayLength=double(4)  InitialCondition=0  InputProcessing=Inherited
  out0 : Outport  OutDataTypeStr=fixdt(1, 24, 14)  InitialOutput=0
  wires:
  in0/1 -> Delay2/1
  Delay2/1 -> out0/1

== system gm_fourxfour_designfxdpt_givens_vnl/fourxfour_designfxdpt/Givens_Boundary_Cell2/Delay3 ==
  in0 : Inport  OutDataTypeStr=fixdt(1, 24, 14)  SampleTime=1e-08
  Enable_out6 : EnablePort  OutDataTypeStr=boolean
  Delay3 : Delay  DelayLength=double(4)  InitialCondition=0  InputProcessing=Inherited
  out0 : Outport  OutDataTypeStr=fixdt(1, 24, 14)  InitialOutput=0
  wires:
  in0/1 -> Delay3/1
  Delay3/1 -> out0/1

== system gm_fourxfour_designfxdpt_givens_vnl/fourxfour_designfxdpt/Givens_Boundary_Cell2/Delay4 ==
  in0 : Inport  OutDataTypeStr=fixdt(0, 49, 28)  SampleTime=1e-08
  Enable_out6 : EnablePort  OutDataTypeStr=boolean
  Delay4 : Delay  DelayLength=double(5)  InitialCondition=0  InputProcessing=Inherited
  out0 : Outport  OutDataTypeStr=fixdt(0, 49, 28)  InitialOutput=0
  wires:
  in0/1 -> Delay4/1
  Delay4/1 -> out0/1

== system gm_fourxfour_designfxdpt_givens_vnl/fourxfour_designfxdpt/Givens_Boundary_Cell2/Delay5 ==
  in0 : Inport  OutDataTypeStr=fixdt(1, 73, 34)  SampleTime=1e-08
  Enable_out6 : EnablePort  OutDataTypeStr=boolean
  Delay5 : Delay  DelayLength=double(4)  InitialCondition=0  InputProcessing=Inherited
  out0 : Outport  OutDataTypeStr=fixdt(1, 73, 34)  InitialOutput=0
  wires:
  in0/1 -> Delay5/1
  Delay5/1 -> out0/1

== system gm_fourxfour_designfxdpt_givens_vnl/fourxfour_designfxdpt/Givens_Boundary_Cell2/Delay6 ==
  in0 : Inport  OutDataTypeStr=fixdt(1, 73, 34)  SampleTime=1e-08
  Enable_out6 : EnablePort  OutDataTypeStr=boolean
  Delay6 : Delay  DelayLength=double(4)  InitialCondition=0  InputProcessing=Inherited
  out0 : Outport  OutDataTypeStr=fixdt(1, 73, 34)  InitialOutput=0
  wires:
  in0/1 -> Delay6/1
  Delay6/1 -> out0/1

== system gm_fourxfour_designfxdpt_givens_vnl/fourxfour_designfxdpt/Givens_Boundary_Cell2/HDL Reciprocal ==
  In1 : Inport
  Delay1 : Delay  DelayLength=1  InputProcessing=Inherited
  Delay2 : Delay  DelayLength=3  InputProcessing=Inherited
  HDL Reciprocal : Reciprocal  SampleTime=1e-08
  Out1 : Outport
  wires:
  Delay2/1 -> Out1/1
  HDL Reciprocal/1 -> Delay2/1
  Delay1/1 -> HDL Reciprocal/1
  In1/1 -> Delay1/1

== system gm_fourxfour_designfxdpt_givens_vnl/fourxfour_designfxdpt/Givens_Boundary_Cell3/Delay1 ==
  in0 : Inport  OutDataTypeStr=fixdt(1, 48, 28)  SampleTime=1e-08
  Enable_out6 : EnablePort  OutDataTypeStr=boolean
  Delay1 : Delay  DelayLength=double(1)  InitialCondition=0  InputProcessing=Inherited
  out0 : Outport  OutDataTypeStr=fixdt(1, 48, 28)  InitialOutput=0
  wires:
  in0/1 -> Delay1/1
  Delay1/1 -> out0/1

== system gm_fourxfour_designfxdpt_givens_vnl/fourxfour_designfxdpt/Givens_Boundary_Cell3/Delay2 ==
  in0 : Inport  OutDataTypeStr=fixdt(1, 24, 14)  SampleTime=1e-08
  Enable_out6 : EnablePort  OutDataTypeStr=boolean
  Delay2 : Delay  DelayLength=double(4)  InitialCondition=0  InputProcessing=Inherited
  out0 : Outport  OutDataTypeStr=fixdt(1, 24, 14)  InitialOutput=0
  wires:
  in0/1 -> Delay2/1
  Delay2/1 -> out0/1

== system gm_fourxfour_designfxdpt_givens_vnl/fourxfour_designfxdpt/Givens_Boundary_Cell3/Delay3 ==
  in0 : Inport  OutDataTypeStr=fixdt(1, 24, 14)  SampleTime=1e-08
  Enable_out6 : EnablePort  OutDataTypeStr=boolean
  Delay3 : Delay  DelayLength=double(4)  InitialCondition=0  InputProcessing=Inherited
  out0 : Outport  OutDataTypeStr=fixdt(1, 24, 14)  InitialOutput=0
  wires:
  in0/1 -> Delay3/1
  Delay3/1 -> out0/1

== system gm_fourxfour_designfxdpt_givens_vnl/fourxfour_designfxdpt/Givens_Boundary_Cell3/Delay4 ==
  in0 : Inport  OutDataTypeStr=fixdt(0, 49, 28)  SampleTime=1e-08
  Enable_out6 : EnablePort  OutDataTypeStr=boolean
  Delay4 : Delay  DelayLength=double(5)  InitialCondition=0  InputProcessing=Inherited
  out0 : Outport  OutDataTypeStr=fixdt(0, 49, 28)  InitialOutput=0
  wires:
  in0/1 -> Delay4/1
  Delay4/1 -> out0/1

== system gm_fourxfour_designfxdpt_givens_vnl/fourxfour_designfxdpt/Givens_Boundary_Cell3/Delay5 ==
  in0 : Inport  OutDataTypeStr=fixdt(1, 73, 34)  SampleTime=1e-08
  Enable_out6 : EnablePort  OutDataTypeStr=boolean
  Delay5 : Delay  DelayLength=double(4)  InitialCondition=0  InputProcessing=Inherited
  out0 : Outport  OutDataTypeStr=fixdt(1, 73, 34)  InitialOutput=0
  wires:
  in0/1 -> Delay5/1
  Delay5/1 -> out0/1

== system gm_fourxfour_designfxdpt_givens_vnl/fourxfour_designfxdpt/Givens_Boundary_Cell3/Delay6 ==
  in0 : Inport  OutDataTypeStr=fixdt(1, 73, 34)  SampleTime=1e-08
  Enable_out6 : EnablePort  OutDataTypeStr=boolean
  Delay6 : Delay  DelayLength=double(4)  InitialCondition=0  InputProcessing=Inherited
  out0 : Outport  OutDataTypeStr=fixdt(1, 73, 34)  InitialOutput=0
  wires:
  in0/1 -> Delay6/1
  Delay6/1 -> out0/1

== system gm_fourxfour_designfxdpt_givens_vnl/fourxfour_designfxdpt/Givens_Boundary_Cell3/HDL Reciprocal ==
  In1 : Inport
  Delay1 : Delay  DelayLength=1  InputProcessing=Inherited
  Delay2 : Delay  DelayLength=3  InputProcessing=Inherited
  HDL Reciprocal : Reciprocal  SampleTime=1e-08
  Out1 : Outport
  wires:
  Delay2/1 -> Out1/1
  HDL Reciprocal/1 -> Delay2/1
  Delay1/1 -> HDL Reciprocal/1
  In1/1 -> Delay1/1

== system gm_fourxfour_designfxdpt_givens_vnl/fourxfour_designfxdpt/Givens_Internal_BW_Cell/Delay ==
  in0 : Inport  OutDataTypeStr=fixdt(1, 24, 14)  SampleTime=1e-08
  Enable_out6 : EnablePort  OutDataTypeStr=boolean
  Delay : Delay  DelayLength=double(1)  InitialCondition=0  InputProcessing=Inherited
  out0 : Outport  OutDataTypeStr=fixdt(1, 24, 14)  InitialOutput=0
  wires:
  in0/1 -> Delay/1
  Delay/1 -> out0/1

== system gm_fourxfour_designfxdpt_givens_vnl/fourxfour_designfxdpt/Givens_Internal_BW_Cell/Delay1 ==
  in0 : Inport  OutDataTypeStr=fixdt(1, 24, 14)  SampleTime=1e-08
  Enable_out6 : EnablePort  OutDataTypeStr=boolean
  Delay1 : Delay  DelayLength=double(1)  InitialCondition=0  InputProcessing=Inherited
  out0 : Outport  OutDataTypeStr=fixdt(1, 24, 14)  InitialOutput=0
  wires:
  in0/1 -> Delay1/1
  Delay1/1 -> out0/1

== system gm_fourxfour_designfxdpt_givens_vnl/fourxfour_designfxdpt/Givens_Internal_BW_Cell/complex_mul ==
  In1_r : Inport  OutDataTypeStr=fixdt(1, 24, 14)  PortDimensions=1  SampleTime=1e-08
  In1_i : Inport  Port=2  OutDataTypeStr=fixdt(1, 24, 14)  PortDimensions=1  SampleTime=1e-08
  In2_r : Inport  Port=3  OutDataTypeStr=fixdt(1, 24, 14)  PortDimensions=1  SampleTime=1e-08
  In2_i : Inport  Port=4  OutDataTypeStr=fixdt(1, 24, 14)  PortDimensions=1  SampleTime=1e-08
  Add : Sum  Inputs=+-
  Add1 : Sum
  Product{,1..3} (4 alike) : Product
  Out1_r : Outport  InitialOutput=0
  Out1_i : Outport  Port=2  InitialOutput=0
  wires:
  Product3/1 -> Add1/2
  Product2/1 -> Add1/1
  Product1/1 -> Add/2
  Product/1 -> Add/1
  Add1/1 -> Out1_i/1
  Add/1 -> Out1_r/1
  In2_i/1 -> Product1/2, Product3/2
  In2_r/1 -> Product/2, Product2/2
  In1_i/1 -> Product1/1, Product2/1
  In1_r/1 -> Product/1, Product3/1

== system gm_fourxfour_designfxdpt_givens_vnl/fourxfour_designfxdpt/Givens_Internal_BW_Cell/complex_mul1 ==
  In1_r : Inport  OutDataTypeStr=fixdt(1, 24, 14)  PortDimensions=1  SampleTime=1e-08
  In1_i : Inport  Port=2  OutDataTypeStr=fixdt(1, 24, 14)  PortDimensions=1  SampleTime=1e-08
  In2_r : Inport  Port=3  OutDataTypeStr=fixdt(1, 24, 14)  PortDimensions=1  SampleTime=1e-08
  In2_i : Inport  Port=4  OutDataTypeStr=fixdt(1, 24, 14)  PortDimensions=1  SampleTime=1e-08
  Add : Sum  Inputs=+-
  Add1 : Sum
  Product{,1..3} (4 alike) : Product
  Out1_r : Outport  InitialOutput=0
  Out1_i : Outport  Port=2  InitialOutput=0
  wires:
  Product3/1 -> Add1/2
  Product2/1 -> Add1/1
  Product1/1 -> Add/2
  Product/1 -> Add/1
  Add1/1 -> Out1_i/1
  Add/1 -> Out1_r/1
  In2_i/1 -> Product1/2, Product3/2
  In2_r/1 -> Product/2, Product2/2
  In1_i/1 -> Product1/1, Product2/1
  In1_r/1 -> Product/1, Product3/1

== system gm_fourxfour_designfxdpt_givens_vnl/fourxfour_designfxdpt/Givens_Internal_BW_Cell1/Delay ==
  in0 : Inport  OutDataTypeStr=fixdt(1, 24, 14)  SampleTime=1e-08
  Enable_out6 : EnablePort  OutDataTypeStr=boolean
  Delay : Delay  DelayLength=double(1)  InitialCondition=0  InputProcessing=Inherited
  out0 : Outport  OutDataTypeStr=fixdt(1, 24, 14)  InitialOutput=0
  wires:
  in0/1 -> Delay/1
  Delay/1 -> out0/1

== system gm_fourxfour_designfxdpt_givens_vnl/fourxfour_designfxdpt/Givens_Internal_BW_Cell1/Delay1 ==
  in0 : Inport  OutDataTypeStr=fixdt(1, 24, 14)  SampleTime=1e-08
  Enable_out6 : EnablePort  OutDataTypeStr=boolean
  Delay1 : Delay  DelayLength=double(1)  InitialCondition=0  InputProcessing=Inherited
  out0 : Outport  OutDataTypeStr=fixdt(1, 24, 14)  InitialOutput=0
  wires:
  in0/1 -> Delay1/1
  Delay1/1 -> out0/1

== system gm_fourxfour_designfxdpt_givens_vnl/fourxfour_designfxdpt/Givens_Internal_BW_Cell1/complex_mul ==
  In1_r : Inport  OutDataTypeStr=fixdt(1, 24, 14)  PortDimensions=1  SampleTime=1e-08
  In1_i : Inport  Port=2  OutDataTypeStr=fixdt(1, 24, 14)  PortDimensions=1  SampleTime=1e-08
  In2_r : Inport  Port=3  OutDataTypeStr=fixdt(1, 24, 14)  PortDimensions=1  SampleTime=1e-08
  In2_i : Inport  Port=4  OutDataTypeStr=fixdt(1, 24, 14)  PortDimensions=1  SampleTime=1e-08
  Add : Sum  Inputs=+-
  Add1 : Sum
  Product{,1..3} (4 alike) : Product
  Out1_r : Outport  InitialOutput=0
  Out1_i : Outport  Port=2  InitialOutput=0
  wires:
  Product3/1 -> Add1/2
  Product2/1 -> Add1/1
  Product1/1 -> Add/2
  Product/1 -> Add/1
  Add1/1 -> Out1_i/1
  Add/1 -> Out1_r/1
  In2_i/1 -> Product1/2, Product3/2
  In2_r/1 -> Product/2, Product2/2
  In1_i/1 -> Product1/1, Product2/1
  In1_r/1 -> Product/1, Product3/1

== system gm_fourxfour_designfxdpt_givens_vnl/fourxfour_designfxdpt/Givens_Internal_BW_Cell1/complex_mul1 ==
  In1_r : Inport  OutDataTypeStr=fixdt(1, 24, 14)  PortDimensions=1  SampleTime=1e-08
  In1_i : Inport  Port=2  OutDataTypeStr=fixdt(1, 24, 14)  PortDimensions=1  SampleTime=1e-08
  In2_r : Inport  Port=3  OutDataTypeStr=fixdt(1, 24, 14)  PortDimensions=1  SampleTime=1e-08
  In2_i : Inport  Port=4  OutDataTypeStr=fixdt(1, 24, 14)  PortDimensions=1  SampleTime=1e-08
  Add : Sum  Inputs=+-
  Add1 : Sum
  Product{,1..3} (4 alike) : Product
  Out1_r : Outport  InitialOutput=0
  Out1_i : Outport  Port=2  InitialOutput=0
  wires:
  Product3/1 -> Add1/2
  Product2/1 -> Add1/1
  Product1/1 -> Add/2
  Product/1 -> Add/1
  Add1/1 -> Out1_i/1
  Add/1 -> Out1_r/1
  In2_i/1 -> Product1/2, Product3/2
  In2_r/1 -> Product/2, Product2/2
  In1_i/1 -> Product1/1, Product2/1
  In1_r/1 -> Product/1, Product3/1

== system gm_fourxfour_designfxdpt_givens_vnl/fourxfour_designfxdpt/Givens_Internal_BW_Cell2/Delay ==
  in0 : Inport  OutDataTypeStr=fixdt(1, 24, 14)  SampleTime=1e-08
  Enable_out6 : EnablePort  OutDataTypeStr=boolean
  Delay : Delay  DelayLength=double(1)  InitialCondition=0  InputProcessing=Inherited
  out0 : Outport  OutDataTypeStr=fixdt(1, 24, 14)  InitialOutput=0
  wires:
  in0/1 -> Delay/1
  Delay/1 -> out0/1

== system gm_fourxfour_designfxdpt_givens_vnl/fourxfour_designfxdpt/Givens_Internal_BW_Cell2/Delay1 ==
  in0 : Inport  OutDataTypeStr=fixdt(1, 24, 14)  SampleTime=1e-08
  Enable_out6 : EnablePort  OutDataTypeStr=boolean
  Delay1 : Delay  DelayLength=double(1)  InitialCondition=0  InputProcessing=Inherited
  out0 : Outport  OutDataTypeStr=fixdt(1, 24, 14)  InitialOutput=0
  wires:
  in0/1 -> Delay1/1
  Delay1/1 -> out0/1

== system gm_fourxfour_designfxdpt_givens_vnl/fourxfour_designfxdpt/Givens_Internal_BW_Cell2/complex_mul ==
  In1_r : Inport  OutDataTypeStr=fixdt(1, 24, 14)  PortDimensions=1  SampleTime=1e-08
  In1_i : Inport  Port=2  OutDataTypeStr=fixdt(1, 24, 14)  PortDimensions=1  SampleTime=1e-08
  In2_r : Inport  Port=3  OutDataTypeStr=fixdt(1, 24, 14)  PortDimensions=1  SampleTime=1e-08
  In2_i : Inport  Port=4  OutDataTypeStr=fixdt(1, 24, 14)  PortDimensions=1  SampleTime=1e-08
  Add : Sum  Inputs=+-
  Add1 : Sum
  Product{,1..3} (4 alike) : Product
  Out1_r : Outport  InitialOutput=0
  Out1_i : Outport  Port=2  InitialOutput=0
  wires:
  Product3/1 -> Add1/2
  Product2/1 -> Add1/1
  Product1/1 -> Add/2
  Product/1 -> Add/1
  Add1/1 -> Out1_i/1
  Add/1 -> Out1_r/1
  In2_i/1 -> Product1/2, Product3/2
  In2_r/1 -> Product/2, Product2/2
  In1_i/1 -> Product1/1, Product2/1
  In1_r/1 -> Product/1, Product3/1

== system gm_fourxfour_designfxdpt_givens_vnl/fourxfour_designfxdpt/Givens_Internal_BW_Cell2/complex_mul1 ==
  In1_r : Inport  OutDataTypeStr=fixdt(1, 24, 14)  PortDimensions=1  SampleTime=1e-08
  In1_i : Inport  Port=2  OutDataTypeStr=fixdt(1, 24, 14)  PortDimensions=1  SampleTime=1e-08
  In2_r : Inport  Port=3  OutDataTypeStr=fixdt(1, 24, 14)  PortDimensions=1  SampleTime=1e-08
  In2_i : Inport  Port=4  OutDataTypeStr=fixdt(1, 24, 14)  PortDimensions=1  SampleTime=1e-08
  Add : Sum  Inputs=+-
  Add1 : Sum
  Product{,1..3} (4 alike) : Product
  Out1_r : Outport  InitialOutput=0
  Out1_i : Outport  Port=2  InitialOutput=0
  wires:
  Product3/1 -> Add1/2
  Product2/1 -> Add1/1
  Product1/1 -> Add/2
  Product/1 -> Add/1
  Add1/1 -> Out1_i/1
  Add/1 -> Out1_r/1
  In2_i/1 -> Product1/2, Product3/2
  In2_r/1 -> Product/2, Product2/2
  In1_i/1 -> Product1/1, Product2/1
  In1_r/1 -> Product/1, Product3/1

== system gm_fourxfour_designfxdpt_givens_vnl/fourxfour_designfxdpt/Givens_Internal_BW_Cell3/Delay ==
  in0 : Inport  OutDataTypeStr=fixdt(1, 24, 14)  SampleTime=1e-08
  Enable_out6 : EnablePort  OutDataTypeStr=boolean
  Delay : Delay  DelayLength=double(1)  InitialCondition=0  InputProcessing=Inherited
  out0 : Outport  OutDataTypeStr=fixdt(1, 24, 14)  InitialOutput=0
  wires:
  in0/1 -> Delay/1
  Delay/1 -> out0/1

== system gm_fourxfour_designfxdpt_givens_vnl/fourxfour_designfxdpt/Givens_Internal_BW_Cell3/Delay1 ==
  in0 : Inport  OutDataTypeStr=fixdt(1, 24, 14)  SampleTime=1e-08
  Enable_out6 : EnablePort  OutDataTypeStr=boolean
  Delay1 : Delay  DelayLength=double(1)  InitialCondition=0  InputProcessing=Inherited
  out0 : Outport  OutDataTypeStr=fixdt(1, 24, 14)  InitialOutput=0
  wires:
  in0/1 -> Delay1/1
  Delay1/1 -> out0/1

== system gm_fourxfour_designfxdpt_givens_vnl/fourxfour_designfxdpt/Givens_Internal_BW_Cell3/complex_mul ==
  In1_r : Inport  OutDataTypeStr=fixdt(1, 24, 14)  PortDimensions=1  SampleTime=1e-08
  In1_i : Inport  Port=2  OutDataTypeStr=fixdt(1, 24, 14)  PortDimensions=1  SampleTime=1e-08
  In2_r : Inport  Port=3  OutDataTypeStr=fixdt(1, 24, 14)  PortDimensions=1  SampleTime=1e-08
  In2_i : Inport  Port=4  OutDataTypeStr=fixdt(1, 24, 14)  PortDimensions=1  SampleTime=1e-08
  Add : Sum  Inputs=+-
  Add1 : Sum
  Product{,1..3} (4 alike) : Product
  Out1_r : Outport  InitialOutput=0
  Out1_i : Outport  Port=2  InitialOutput=0
  wires:
  Product3/1 -> Add1/2
  Product2/1 -> Add1/1
  Product1/1 -> Add/2
  Product/1 -> Add/1
  Add1/1 -> Out1_i/1
  Add/1 -> Out1_r/1
  In2_i/1 -> Product1/2, Product3/2
  In2_r/1 -> Product/2, Product2/2
  In1_i/1 -> Product1/1, Product2/1
  In1_r/1 -> Product/1, Product3/1

== system gm_fourxfour_designfxdpt_givens_vnl/fourxfour_designfxdpt/Givens_Internal_BW_Cell3/complex_mul1 ==
  In1_r : Inport  OutDataTypeStr=fixdt(1, 24, 14)  PortDimensions=1  SampleTime=1e-08
  In1_i : Inport  Port=2  OutDataTypeStr=fixdt(1, 24, 14)  PortDimensions=1  SampleTime=1e-08
  In2_r : Inport  Port=3  OutDataTypeStr=fixdt(1, 24, 14)  PortDimensions=1  SampleTime=1e-08
  In2_i : Inport  Port=4  OutDataTypeStr=fixdt(1, 24, 14)  PortDimensions=1  SampleTime=1e-08
  Add : Sum  Inputs=+-
  Add1 : Sum
  Product{,1..3} (4 alike) : Product
  Out1_r : Outport  InitialOutput=0
  Out1_i : Outport  Port=2  InitialOutput=0
  wires:
  Product3/1 -> Add1/2
  Product2/1 -> Add1/1
  Product1/1 -> Add/2
  Product/1 -> Add/1
  Add1/1 -> Out1_i/1
  Add/1 -> Out1_r/1
  In2_i/1 -> Product1/2, Product3/2
  In2_r/1 -> Product/2, Product2/2
  In1_i/1 -> Product1/1, Product2/1
  In1_r/1 -> Product/1, Product3/1

== system gm_fourxfour_designfxdpt_givens_vnl/fourxfour_designfxdpt/Givens_Internal_QR_Cell/Delay ==
  in0 : Inport  OutDataTypeStr=fixdt(1, 24, 14)  SampleTime=1e-08
  Enable_out11 : EnablePort  OutDataTypeStr=boolean
  Delay : Delay  DelayLength=double(1)  InitialCondition=0  InputProcessing=Inherited
  out0 : Outport  OutDataTypeStr=fixdt(1, 24, 14)  InitialOutput=0
  wires:
  in0/1 -> Delay/1
  Delay/1 -> out0/1

== system gm_fourxfour_designfxdpt_givens_vnl/fourxfour_designfxdpt/Givens_Internal_QR_Cell/Delay1 ==
  in0 : Inport  OutDataTypeStr=fixdt(1, 24, 14)  SampleTime=1e-08
  Enable_out11 : EnablePort  OutDataTypeStr=boolean
  Delay1 : Delay  DelayLength=double(1)  InitialCondition=0  InputProcessing=Inherited
  out0 : Outport  OutDataTypeStr=fixdt(1, 24, 14)  InitialOutput=0
  wires:
  in0/1 -> Delay1/1
  Delay1/1 -> out0/1

== system gm_fourxfour_designfxdpt_givens_vnl/fourxfour_designfxdpt/Givens_Internal_QR_Cell/complex_mul ==
  In1_r : Inport  OutDataTypeStr=fixdt(1, 24, 14)  PortDimensions=1  SampleTime=1e-08
  In1_i : Inport  Port=2  OutDataTypeStr=fixdt(1, 24, 14)  PortDimensions=1  SampleTime=1e-08
  In2_r : Inport  Port=3  OutDataTypeStr=fixdt(1, 24, 14)  PortDimensions=1  SampleTime=1e-08
  In2_i : Inport  Port=4  OutDataTypeStr=fixdt(1, 24, 14)  PortDimensions=1  SampleTime=1e-08
  Add : Sum  Inputs=+-
  Add1 : Sum
  Product{,1..3} (4 alike) : Product
  Out1_r : Outport  InitialOutput=0
  Out1_i : Outport  Port=2  InitialOutput=0
  wires:
  Product3/1 -> Add1/2
  Product2/1 -> Add1/1
  Product1/1 -> Add/2
  Product/1 -> Add/1
  Add1/1 -> Out1_i/1
  Add/1 -> Out1_r/1
  In2_i/1 -> Product1/2, Product3/2
  In2_r/1 -> Product/2, Product2/2
  In1_i/1 -> Product1/1, Product2/1
  In1_r/1 -> Product/1, Product3/1

== system gm_fourxfour_designfxdpt_givens_vnl/fourxfour_designfxdpt/Givens_Internal_QR_Cell/complex_mul1 ==
  In1_r : Inport  OutDataTypeStr=fixdt(1, 24, 14)  PortDimensions=1  SampleTime=1e-08
  In1_i : Inport  Port=2  OutDataTypeStr=fixdt(1, 24, 14)  PortDimensions=1  SampleTime=1e-08
  In2_r : Inport  Port=3  OutDataTypeStr=fixdt(1, 24, 14)  PortDimensions=1  SampleTime=1e-08
  In2_i : Inport  Port=4  OutDataTypeStr=fixdt(1, 24, 14)  PortDimensions=1  SampleTime=1e-08
  Add : Sum  Inputs=+-
  Add1 : Sum
  Product{,1..3} (4 alike) : Product
  Out1_r : Outport  InitialOutput=0
  Out1_i : Outport  Port=2  InitialOutput=0
  wires:
  Product3/1 -> Add1/2
  Product2/1 -> Add1/1
  Product1/1 -> Add/2
  Product/1 -> Add/1
  Add1/1 -> Out1_i/1
  Add/1 -> Out1_r/1
  In2_i/1 -> Product1/2, Product3/2
  In2_r/1 -> Product/2, Product2/2
  In1_i/1 -> Product1/1, Product2/1
  In1_r/1 -> Product/1, Product3/1

== system gm_fourxfour_designfxdpt_givens_vnl/fourxfour_designfxdpt/Givens_Internal_QR_Cell/complex_mul_rz1 ==
  In1_r : Inport  OutDataTypeStr=fixdt(1, 24, 14)  PortDimensions=1  SampleTime=1e-08
  In1_i : Inport  Port=2  OutDataTypeStr=fixdt(1, 24, 14)  PortDimensions=1  SampleTime=1e-08
  In2_r : Inport  Port=3  OutDataTypeStr=fixdt(1, 24, 14)  PortDimensions=1  SampleTime=1e-08
  In2_i : Inport  Port=4  OutDataTypeStr=fixdt(1, 24, 14)  PortDimensions=1  SampleTime=1e-08
  Add : Sum  Inputs=+-
  Add1 : Sum
  Data Type Conversion{1..3,13} (4 alike) : DataTypeConversion  OutDataTypeStr=data1
  Product{,1..3} (4 alike) : Product
  Out1_r : Outport  InitialOutput=0
  Out1_i : Outport  Port=2  InitialOutput=0
  wires:
  Product3/1 -> Data Type Conversion3/1
  Product2/1 -> Data Type Conversion2/1
  Product1/1 -> Data Type Conversion1/1
  Product/1 -> Data Type Conversion13/1
  Data Type Conversion3/1 -> Add1/2
  Data Type Conversion2/1 -> Add1/1
  Data Type Conversion13/1 -> Add/1
  Data Type Conversion1/1 -> Add/2
  Add1/1 -> Out1_i/1
  Add/1 -> Out1_r/1
  In2_i/1 -> Product1/2, Product3/2
  In2_r/1 -> Product/2, Product2/2
  In1_i/1 -> Product1/1, Product2/1
  In1_r/1 -> Product/1, Product3/1

== system gm_fourxfour_designfxdpt_givens_vnl/fourxfour_designfxdpt/Givens_Internal_QR_Cell1/Delay ==
  in0 : Inport  OutDataTypeStr=fixdt(1, 24, 14)  SampleTime=1e-08
  Enable_out11 : EnablePort  OutDataTypeStr=boolean
  Delay : Delay  DelayLength=double(1)  InitialCondition=0  InputProcessing=Inherited
  out0 : Outport  OutDataTypeStr=fixdt(1, 24, 14)  InitialOutput=0
  wires:
  in0/1 -> Delay/1
  Delay/1 -> out0/1
